simulink library "tqd"  (R2021b)
settings: Solver=VariableStepAuto  StartTime=0.0  StopTime=10.0  RelTol=1e-3
undefined symbols (not defined in the file or in its folder): ATQD_APSDecReq_X_kph, ATQD_APSDecReq_Y_mps2, ATQD_APSDecReqCMD_X_kph, ATQD_APSDecReqTs_X_pct, ATQD_APSDecTimeGain_X_Deg, ATQD_APSDecTimeGain_Y_s, ATQD_APSReqLowSpd_X_Deg, ATQD_AutoHoldReleaseBPS_X_Deg, ATQD_AWDLoadTrqnsGain_X_kg, ATQD_AWDLoadTrqnsGain_Y_pct, ATQD_BOSEnBPSPosn_X_kph, ATQD_BOSMap_X_rpm, ATQD_BOSMap_Y_pct, ATQD_CreepBaseTqD_X_kph, ATQD_CreepBaseTqD_Y_Deg, ATQD_CreepBaseTqR_X_kph, ATQD_CreepBaseTqR_Y_Deg, ATQD_CreepBPSDisPosn_X_Deg, ATQD_CreepBPSDisPosnR_X_Deg, ATQD_CreepBPSEnPosn_X_Deg, ATQD_CreepBPSEnPosnR_X_Deg, ATQD_CreepDeltaTq_X_kph, ATQD_CreepIterm_X_kph, ATQD_CreepIterm_Y_kph, ATQD_CreepItermMaxLimit_X_pct, ATQD_CreepPreloadTime_X_kph, ATQD_CreepPreloadTq_X_kph, ATQD_CreepPreloadTq_Y_s, ATQD_CreepProtTq_X_Deg, ATQD_CreepPterm_X_kph, ATQD_CreepPterm_Y_kph, ATQD_ECOTqMapD_X_rpm, ATQD_ECOTqMapD_Y_pct, ATQD_EOPDTqMapDCon_X_rpm, ATQD_EOPDTqMapDCon_Y_Deg, ATQD_EstInitVehWeight_X_c, ATQD_LHMRollGenMapD_X_rpm, ATQD_LHMRollGenMapD_Y_rpm, ATQD_LHMTqMapD_X_rpm, ATQD_LHMTqMapD_Y_pct, ATQD_NL1TqMapD_X_rpm, ATQD_NL1TqMapD_Y_pct, ATQD_NOPDTqMapDCon_X_rpm, ATQD_NOPDTqMapDCon_Y_Deg, ATQD_NRMRrEDUSpRat_X_rpm, ATQD_NRMRrEDUSpRat_Y_Nm, ATQD_OPDHoldDownRelDelay_X_Deg, ATQD_OPDHoldEnSpd_X_Deg, ATQD_OPDHoldRelDetTime_X_Deg, ATQD_OPDHoldReleaseTq_X_Deg, ATQD_OrigPedTqLowLim_X_Deg, ATQD_OrigPedTqLowLim_Y_pct, ATQD_PedalMapClimbUpLim_X_rpm, ATQD_PedalMapClimbUpLim_Y_Deg, ATQD_PreLoadTq_X_s, ATQD_RollGenMapEL1_X_rpm, ATQD_RollGenMapEL1_Y_rpm, ATQD_SL1TqMapD_X_rpm, ATQD_SL1TqMapD_Y_pct, ATQD_SlideRegenTqGain_X_Gps ... (+491)
libraries: hcu_lib x83, simulink x73, tqr x1
(part 3 of 19)

== system tqd/TQD/TorqueDemand/CrashDetect ==
  VPMM_PowerSta_enum : Inport
  VINP_CrashSignalGPIO_flg : Inport  Port=2
  VINP_CrashOutputSts_enum : Inport  Port=3
  task_time_s : Inport  Port=4
  Add1 : Sum
  Add2 : Sum
  Add3 : Sum
  Constant1 : Constant  Value=ENUM_POWERSTA_ON
  Constant{3,8,10,19,23,36} (6 alike) : Constant  Value=KTQD_CrashPWMCnt_cnt
  Constant{6,11,20,26,31,34} (6 alike) : Constant  Value=ZERO_INT
  Constant12 : Constant  Value=KTQD_50MS_cnt
  Constant13 : Constant  Value=KTQD_PwrStaTimerforCrash_s
  Constant14 : Constant  Value=ENUM_CRASHSTATE_NOCRASH
  Constant15 : Constant  Value=KTQD_DiagHCrashTimer_s
  Constant16 : Constant  Value=ENUM_CRASHSTATE_NOCRASH
  Constant17 : Constant  Value=ENUM_CRASHSTATE_NOCRASH
  Constant18 : Constant  Value=KTQD_PwrStaTimerforCrash_s
  Constant2 : Constant  Value=ENUM_POWERSTA_READY
  Constant21 : Constant  Value=KTQD_50MS_cnt
  Constant22 : Constant  Value=ZERO_FLOAT
  Constant24 : Constant  Value=KTQD_NoDiagHCrashTimer_s
  Constant25 : Constant  Value=KTQD_DiagHCrashTimer_s
  Constant27 : Constant  Value=KTQD_190MS_cnt
  Constant28 : Constant  Value=KTQD_30MS_cnt
  Constant29 : Constant  Value=KTQD_50MS_cnt
  Constant30 : Constant  Value=KTQD_210MS_cnt
  Constant32 : Constant  Value=KTQD_NoDiagHCrashTimer_s
  Constant35 : Constant  Value=KTQD_210MS_cnt
  Constant4 : Constant  Value=ONE_INT
  Constant5 : Constant  Value=ENUM_POWERSTA_OFF
  Constant7 : Constant  Value=KTQD_210MS_cnt
  Constant9 : Constant  Value=FALSE
  Data Type Conversion1 : DataTypeConversion
  Data Type Conversion2 : DataTypeConversion
  Equal : RelationalOperator  Operator=~=  OutDataTypeStr=boolean  RndMeth=Simplest
  Equal{1..2,6,10} (4 alike) : RelationalOperator  Operator===  OutDataTypeStr=boolean  RndMeth=Simplest
  Equal{3,7,9,11,13} (5 alike) : RelationalOperator  OutDataTypeStr=boolean  RndMeth=Simplest
  Equal12 : RelationalOperator  Operator=<  OutDataTypeStr=boolean  RndMeth=Simplest
  Equal4 : RelationalOperator  Operator=~=  OutDataTypeStr=boolean  RndMeth=Simplest
  Equal5 : RelationalOperator  Operator=<  OutDataTypeStr=boolean  RndMeth=Simplest
  Equal8 : RelationalOperator  Operator=~=  OutDataTypeStr=boolean  RndMeth=Simplest
  Logical Operator{,9..10,13,16,21} (6 alike) : Logic  Operator=OR  AllPortsSameDT=off  OutDataTypeStr=boolean
  Logical Operator{1,3,7..8,18,20} (6 alike) : Logic  Operator=NOT  AllPortsSameDT=off  OutDataTypeStr=boolean
  Logical Operator{4..5,11..12,14..15,17,19} (8 alike) : Logic  AllPortsSameDT=off  OutDataTypeStr=boolean
  Logical Operator2 : Logic  Inputs=3  AllPortsSameDT=off  OutDataTypeStr=boolean
  Logical Operator6 : Logic  Inputs=3  AllPortsSameDT=off  OutDataTypeStr=boolean
  Relational Operator{,5..7,9} (5 alike) : RelationalOperator  Operator=>  OutDataTypeStr=boolean  RndMeth=Simplest
  Relational Operator1 : RelationalOperator  OutDataTypeStr=boolean  RndMeth=Simplest
  Relational Operator10 : RelationalOperator  Operator=<  OutDataTypeStr=boolean  RndMeth=Simplest
  Relational Operator2 : RelationalOperator  Operator=<=  OutDataTypeStr=boolean  RndMeth=Simplest
  Relational Operator3 : RelationalOperator  OutDataTypeStr=boolean  RndMeth=Simplest
  Relational Operator4 : RelationalOperator  Operator=<=  OutDataTypeStr=boolean  RndMeth=Simplest
  Relational Operator8 : RelationalOperator  Operator=<  OutDataTypeStr=boolean  RndMeth=Simplest
  SR_Latch : hcu_lib/Basic_Blocks/SR_Latch
  Switch1 : Switch  Criteria=u2 ~= 0
  Switch{2..9} (8 alike) : Switch  Criteria=u2 > Threshold
  Timer2 : hcu_lib/Basic_Blocks/Timer
  Timer3 : hcu_lib/Basic_Blocks/Timer
  Timer4 : hcu_lib/Basic_Blocks/Timer
  Unit Delay{1..3,5} (4 alike) : UnitDelay  SampleTime=-1  HasFrameUpgradeWarning=on
  VTQD_CrashDetd_flg : Outport
  VTQD_DiagHCrash_flg : Outport  Port=2
  wires:
  [VPMM_PowerSta_enum] -> Equal2/1
  Logical Operator/1 -> Logical Operator3/1, Timer2/1
  [VPMM_PowerSta_enum] -> Equal1/1
  Constant13/1 -> Equal7/2
  Timer2/1 -> Equal7/1
  Constant18/1 -> Timer2/4
  Logical Operator3/1 -> Timer2/2
  Constant1/1 -> Equal1/2
  Constant2/1 -> Equal2/2
  Equal7/1 -> [VTQD_PwrStaTimerReady_flg]  "VTQD_PwrStaTimerReady_flg"
  [task_time_s] -> Timer2/3
  VPMM_PowerSta_enum/1 -> [VPMM_PowerSta_enum]
  VINP_CrashSignalGPIO_flg/1 -> [VINP_CrashSignalGPIO_flg]
  Equal1/1 -> Logical Operator/1
  Equal2/1 -> Logical Operator/2
  VINP_CrashOutputSts_enum/1 -> [VINP_CrashOutputSts_enum]
  task_time_s/1 -> [task_time_s]
  Data Type Conversion1/1 -> Add3/2
  Constant8/1 -> Relational Operator8/2
  Relational Operator8/1 -> Data Type Conversion1/1
  [VTQD_CrashCountEN_flg] -> Switch6/2
  [VTQD_PwrStaTimerReady_flg] -> Switch7/2
  Constant29/1 -> Relational Operator2/2
  Unit Delay3/1 -> Equal/1
  Constant26/1 -> Switch7/3
  Switch6/1 -> Switch3/1
  Logical Operator10/1 -> [VTQD_CrashCountEN_flg]
  Constant22/1 -> Relational Operator/2
  Add2/1 -> Switch2/3
  [VTQD_CrashChange_flg] -> Switch3/2
  Logical Operator6/1 -> Logical Operator10/2
  Constant28/1 -> Relational Operator1/2
  Logical Operator2/1 -> Logical Operator10/1
  Switch3/1 -> Switch7/1
  Equal/1 -> [VTQD_CrashChange_flg]
  Add3/1 -> Switch6/1
  Relational Operator3/1 -> Logical Operator6/2
  Constant6/1 -> Switch6/3
  Constant4/1 -> Add2/2
  Relational Operator2/1 -> Logical Operator2/3
  Logical Operator1/1 -> Logical Operator2/1
  [VTQD_fCrash_cnt] -> Relational Operator8/1, Add3/1
  Switch2/1 -> Unit Delay1/1
  Unit Delay5/1 -> [VTQD_fCrash_cnt], Equal3/1  "VTQD_fCrash_cnt"
  Relational Operator/1 -> Equal/2, Unit Delay3/1
  [VTQD_CrashChange_flg] -> Switch2/2
  [VINP_CrashSignalGPIO_flg] -> Logical Operator1/1
  [VTQD_CrashCount_enum] -> Relational Operator2/1, Relational Operator1/1
  Relational Operator1/1 -> Logical Operator2/2
  Constant31/1 -> Switch2/1
  [VINP_CrashSignalGPIO_flg] -> Relational Operator/1
  Constant10/1 -> Equal3/2
  [VTQD_PwrStaTimerReady_flg] -> Logical Operator12/2
  Logical Operator12/1 -> Logical Operator13/2, [VTQD_CrashOutputSts_flg]
  Equal4/1 -> Logical Operator12/1
  Constant14/1 -> Equal4/2
  [VINP_CrashOutputSts_enum] -> Equal4/1
  Switch7/1 -> Unit Delay5/1
  Unit Delay1/1 -> [VTQD_CrashCount_enum]
  [VTQD_CrashCount_enum] -> Add2/1
  Logical Operator4/1 -> Logical Operator9/2
  [VTQD_CrashCount_enum] -> Relational Operator6/1
  Relational Operator6/1 -> Logical Operator4/2
  [VINP_CrashSignalGPIO_flg] -> Logical Operator8/1
  Logical Operator5/1 -> Logical Operator9/1
  Constant7/1 -> Relational Operator6/2
  Constant11/1 -> Switch4/1
  Logical Operator8/1 -> Logical Operator4/1
  [VTQD_fCrash_cnt] -> Switch4/3
  [VTQD_CrashCount_enum] -> Relational Operator7/1
  Logical Operator9/1 -> Switch4/2
  Relational Operator7/1 -> Logical Operator5/2
  [VINP_CrashSignalGPIO_flg] -> Logical Operator5/1
  Constant12/1 -> Relational Operator7/2
  Switch4/1 -> Switch3/3
  Equal3/1 -> Logical Operator13/1
  Logical Operator13/1 -> VTQD_CrashDetd_flg/1  "VTQD_CrashDetd_flg"
  [VINP_CrashSignalGPIO_flg] -> Logical Operator6/1
  Relational Operator4/1 -> Logical Operator6/3
  Constant30/1 -> Relational Operator4/2
  Constant27/1 -> Relational Operator3/2
  [VTQD_CrashCount_enum] -> Relational Operator4/1, Relational Operator3/1
  [VINP_CrashSignalGPIO_flg] -> Logical Operator19/1
  Equal12/1 -> Logical Operator17/1
  Unit Delay2/1 -> Equal9/1, Equal12/1, [test_crash_cnt]
  Equal9/1 -> Logical Operator14/1
  [VINP_CrashOutputSts_enum] -> Equal8/1
  Data Type Conversion2/1 -> Add1/2
  [VTQD_CrashChange_flg] -> Switch5/2
  [test_crash_cnt] -> Relational Operator10/1, Add1/1
  Switch9/1 -> Switch5/1
  Logical Operator21/1 -> Switch8/2
  Constant15/1 -> Equal11/2
  Relational Operator5/1 -> Logical Operator15/2
  Equal6/1 -> Switch1/2
  Relational Operator10/1 -> Data Type Conversion2/1
  Constant34/1 -> Switch9/3
  [task_time_s] -> Timer4/3
  Logical Operator17/1 -> Logical Operator16/2
  Constant36/1 -> Relational Operator10/2
  SR_Latch/1 -> VTQD_DiagHCrash_flg/1  "VTQD_DiagHCrash_flg"
  Equal10/1 -> Logical Operator17/2
  Logical Operator20/1 -> Logical Operator15/1
  Constant20/1 -> Switch8/1
  Equal13/1 -> Switch1/3
  Relational Operator9/1 -> Logical Operator19/2
  Constant16/1 -> Equal8/2
  [VTQD_CrashCount_enum] -> Relational Operator9/1
  [VINP_CrashOutputSts_enum] -> Equal10/1
  Switch8/1 -> Switch5/3
  Equal11/1 -> Logical Operator11/2
  Logical Operator19/1 -> Logical Operator21/1
  Constant19/1 -> Equal9/2
  Constant21/1 -> Relational Operator9/2
  Constant17/1 -> Equal10/2
  Logical Operator18/1 -> Timer4/2
  [test_crash_cnt] -> Switch8/3
  Constant3/1 -> Equal5/2
  Logical Operator15/1 -> Logical Operator21/2
  Constant35/1 -> Relational Operator5/2
  Constant32/1 -> Timer4/4
  [VTQD_CrashCountEN_flg] -> Switch9/2
  Constant23/1 -> Equal12/2
  Equal8/1 -> Logical Operator14/2
  Constant24/1 -> Equal13/2
  [VPMM_PowerSta_enum] -> Equal6/1
  Add1/1 -> Switch9/1
  Logical Operator11/1 -> SR_Latch/1
  [VTQD_CrashOutputSts_flg] -> Logical Operator7/1, Timer3/1
  Switch1/1 -> SR_Latch/2
  Timer4/1 -> Equal13/1
  Constant9/1 -> Switch1/1
  [VINP_CrashSignalGPIO_flg] -> Logical Operator20/1
  [VTQD_fCrash_cnt] -> Equal5/1
  Logical Operator7/1 -> Timer3/2
  Switch5/1 -> Unit Delay2/1
  Equal5/1 -> Logical Operator11/1
  [task_time_s] -> Timer3/3
  Constant5/1 -> Equal6/2
  [VTQD_CrashCount_enum] -> Relational Operator5/1
  Constant25/1 -> Timer3/4
  Logical Operator16/1 -> Logical Operator18/1, Timer4/1
  Timer3/1 -> Equal11/1
  Logical Operator14/1 -> Logical Operator16/1

== system tqd/TQD/TorqueDemand/ShiftModule ==
  task_time_s : Inport
  VINP_ShifterHandleCmd_enum : Inport  Port=2
  VINP_VehSpeed_kph : Inport  Port=3
  VTQD_BrkSwSta_flg : Inport  Port=4
  VPMM_PowerSta_enum : Inport  Port=5
  VINP_PBWMotorPos_enum : Inport  Port=6
  VTQD_TMRotateDirction_enum : Inport  Port=7
  VTQD_EPBCarWashMode_flg : Inport  Port=8
  VINP_DrDoorSW_flg : Inport  Port=9
  VVMC_APSShiftPosnReq_enum : Inport  Port=10
  VVMC_APSActive_flg : Inport  Port=11
  VINP_DriverSeatBeltCmd_flg : Inport  Port=12
  VINP_SeatSW_flg : Inport  Port=13
  VINP_ChrgPlugSta_enum : Inport  Port=14
  VTQD_IVIPwrLock_flg : Inport  Port=15
  VTQD_AfterAvailableTqDemFr_Nm : Inport  Port=16
  VTQD_AfterAvailableTqDemRr_Nm : Inport  Port=17
  VTQR_NoABSFEDUWhlTqReq_Nm : Inport  Port=18
  VTQR_NoABSREDUWhlTqReq_Nm : Inport  Port=19
  VINP_DOASta_flg : Inport  Port=20
  VINP_MCPressure_bar : Inport  Port=21
  VTQD_OPDHoldAllowPark_flg : Inport  Port=22
  VINP_CAASSta_enum : Inport  Port=23
  VDDM_VCURAPSErrLv2_flg : Inport  Port=24
  VDDM_VCURAPSErrLv3_flg : Inport  Port=25
  VINP_APSStaSystem_enum : Inport  Port=26
  Constant : Constant  Value=KTQD_VehSpd2P_kph
  Constant1 : Constant  Value=KTQD_PBWTimeout_s
  Constant2 : Constant  Value=KTQD_VehSpdRev_kph
  Constant3 : Constant  Value=KTQD_ShiftInitialTime_s
  Constant4 : Constant  Value=KTQD_RelockWaitTime_s
  Constant5 : Constant  Value=KTQD_ReunlockWaitTime_s
  Constant6 : Constant  Value=ENUM_GEARACTUALPOSN_P
  Constant7 : Constant  Value=ENUM_GEARACTUALPOSN_P
  Data Type Conversion1 : DataTypeConversion
  Data Type Conversion2 : DataTypeConversion
  Data Type Conversion3 : DataTypeConversion  OutDataTypeStr=uint8
  Data Type Conversion4 : DataTypeConversion  OutDataTypeStr=boolean
  Determine_Actual_Gear_Position : Stateflow chart  TreatAsAtomicUnit=on
  Equal : RelationalOperator  Operator===  OutDataTypeStr=boolean  RndMeth=Simplest
  Equal1 : RelationalOperator  Operator=~=  OutDataTypeStr=boolean  RndMeth=Simplest
  GearShiftPosn : Subsystem  Description=GearPosition
  P_Button_State_Judge : Subsystem
  SR_Latch : hcu_lib/Basic_Blocks/SR_Latch
  SR_Latch1 : Subsystem  mask(SR_Latch){}
      mask help: SR latch function.
  VTQD_GearActualPosn_enum : Outport
  VTQD_ParkRequest_flg : Outport  Port=2
  VTQD_PBWLockTO_flg : Outport  Port=3
  VTQD_PBWUnlockTO_flg : Outport  Port=4
  VTQD_PButtonSta_enum : Outport  Port=5
  VTQD_DriveProtRemove_flg : Outport  Port=6
  VTQD_DriveProtEn_flg : Outport  Port=7
  wires:
  VPMM_PowerSta_enum/1 -> [VPMM_PowerSta_enum]
  task_time_s/1 -> [task_time_s]
  VINP_VehSpeed_kph/1 -> [VINP_VehSpeed_kph]
  VTQD_BrkSwSta_flg/1 -> [VTQD_BrkSwSta_flg]
  VTQD_TMRotateDirction_enum/1 -> [VTQD_TMRotateDirction_enum]
  VINP_PBWMotorPos_enum/1 -> [VINP_PBWMotorPos_enum]
  P_Button_State_Judge/1(VTQD_PButtonSta_enum) -> VTQD_PButtonSta_enum/1
  VINP_ShifterHandleCmd_enum/1 -> [VINP_ShifterHandleCmd_enum]
  [VINP_ShifterHandleCmd_enum] -> P_Button_State_Judge/1(VINP_ShifterHandleCmd_enum)
  VTQD_IVIPwrLock_flg/1 -> [VTQD_IVIPwrLock_flg]
  VINP_ChrgPlugSta_enum/1 -> [VINP_ChrgPlugSta_enum]
  VINP_SeatSW_flg/1 -> [VINP_SeatSW_flg]
  VINP_DriverSeatBeltCmd_flg/1 -> [VINP_DriverSeatBeltCmd_flg]
  VVMC_APSActive_flg/1 -> [VVMC_APSActive_flg]
  VVMC_APSShiftPosnReq_enum/1 -> [VVMC_APSShiftPosnReq_enum]
  VINP_DrDoorSW_flg/1 -> [VINP_DrDoorSW_flg]
  VTQD_EPBCarWashMode_flg/1 -> [VTQD_EPBCarWashMode_flg]
  [VTQD_EPBCarWashMode_flg] -> GearShiftPosn/8(VTQD_EPBCarWashMode_flg)
  [VINP_VehSpeed_kph] -> GearShiftPosn/9(VINP_VehSpeed_kph)
  [VINP_ChrgPlugSta_enum] -> GearShiftPosn/10(VINP_ChrgPlugSta_enum)
  GearShiftPosn/3(VTQD_PwrStaAllowDR_flg) -> [VTQD_PwrStaAllowDR_flg]
  [VVMC_APSShiftPosnReq_enum] -> GearShiftPosn/4(VVMC_APSShiftPosnReq_enum)
  [VINP_DrDoorSW_flg] -> GearShiftPosn/3(VINP_DrDoorSW_flg)
  [VINP_ShifterHandleCmd_enum] -> GearShiftPosn/1(VINP_ShifterHandleCmd_enum)
  [VVMC_APSActive_flg] -> GearShiftPosn/5(VVMC_APSActive_flg)
  [VINP_DriverSeatBeltCmd_flg] -> GearShiftPosn/6(VINP_DriverSeatBeltCmd_flg)
  GearShiftPosn/1(VTQD_GearShiftCMD_enum) -> [VTQD_GearShiftCMD_enum]
  [VINP_SeatSW_flg] -> GearShiftPosn/7(VINP_SeatSW_flg)
  [VPMM_PowerSta_enum] -> GearShiftPosn/2(VPMM_PowerSta_enum)
  GearShiftPosn/2(VTQD_PwrStaAllowPN_flg) -> [VTQD_PwrStaAllowPN_flg]
  [VVMC_APSActive_flg] -> Determine_Actual_Gear_Position/16(VVMC_APSActive_flg)
  Data Type Conversion4/1 -> VTQD_ParkRequest_flg/1  "VTQD_ParkRequest_flg"
  Constant6/1 -> Equal/2
  [VTQD_EPBCarWashMode_flg] -> Determine_Actual_Gear_Position/15(VINP_EPBCarWashMode_flg)
  Constant4/1 -> Determine_Actual_Gear_Position/13(KTQD_RelockWaitTime_s)
  Constant2/1 -> Determine_Actual_Gear_Position/10(KTQD_VehSpdRev_kph)
  Data Type Conversion1/1 -> SR_Latch/1
  [VTQD_GearActualPosn_enum] -> Equal1/1
  [VTQD_GearActualPosn_enum] -> Equal/1
  Data Type Conversion2/1 -> SR_Latch1/1(set)
  Determine_Actual_Gear_Position/4(VTQD_ParkRequest_flg) -> Data Type Conversion4/1
  Constant7/1 -> Equal1/2
  Data Type Conversion3/1 -> [VTQD_GearActualPosn_enum], VTQD_GearActualPosn_enum/1  "VTQD_GearActualPosn_enum"
  Constant1/1 -> Determine_Actual_Gear_Position/12(KTQD_PBWTimeout_s)
  Constant5/1 -> Determine_Actual_Gear_Position/14(KTQD_ReunlockWaitTime_s)
  [VTQD_PwrStaAllowPN_flg] -> Determine_Actual_Gear_Position/7(VTQD_PwrStaAllowPN_flg)
  Determine_Actual_Gear_Position/3(VTQD_PBWUnlockTO_flg) -> Data Type Conversion2/1
  Constant/1 -> Determine_Actual_Gear_Position/9(KTQD_VehSpd2P_kph)
  [VTQD_TMRotateDirction_enum] -> Determine_Actual_Gear_Position/8(VTQD_TMRotateDirction_enum)
  SR_Latch1/1(latched) -> VTQD_PBWUnlockTO_flg/1  "VTQD_PBWUnlockTO_flg"
  Equal1/1 -> SR_Latch1/2(reset)
  [VINP_VehSpeed_kph] -> Determine_Actual_Gear_Position/4(VINP_VehSpd_kph)
  [VTQD_PwrStaAllowDR_flg] -> Determine_Actual_Gear_Position/6(VTQD_PwrStaAllowDR_flg)
  Constant3/1 -> Determine_Actual_Gear_Position/11(KTQD_ShiftInitialTime_s)
  [VTQD_GearShiftCMD_enum] -> Determine_Actual_Gear_Position/3(VTQD_GearShiftCMD_enum)
  Equal/1 -> SR_Latch/2
  [task_time_s] -> Determine_Actual_Gear_Position/1(task_time_s)
  [VTQD_BrkSwSta_flg] -> Determine_Actual_Gear_Position/2(VTQD_BrkSwSta_flg)
  Determine_Actual_Gear_Position/2(VTQD_PBWLockTO_flg) -> Data Type Conversion1/1
  Determine_Actual_Gear_Position/1(VTQD_GearActualPosn_enum) -> Data Type Conversion3/1
  [VINP_PBWMotorPos_enum] -> Determine_Actual_Gear_Position/5(VINP_PBWMotorPos_enum)
  SR_Latch/1 -> VTQD_PBWLockTO_flg/1  "VTQD_PBWLockTO_flg"
  [VTQD_GearActualPosn_enum] -> GearShiftPosn/11(VTQD_GearActualPosn_enum)
  [VTQD_AfterAvailableTqDemFr_Nm] -> GearShiftPosn/12(VTQD_AfterAvailableTqDemFr_Nm)
  [VTQR_NoABSREDUWhlTqReq_Nm] -> GearShiftPosn/15(VTQR_NoABSREDUWhlTqReq_Nm)
  [VTQR_NoABSFEDUWhlTqReq_Nm] -> GearShiftPosn/14(VTQR_NoABSFEDUWhlTqReq_Nm)
  [VTQD_AfterAvailableTqDemRr_Nm] -> GearShiftPosn/13(VTQD_AfterAvailableTqDemRr_Nm)
  [task_time_s] -> GearShiftPosn/16(task_time_s)
  VTQD_AfterAvailableTqDemFr_Nm/1 -> [VTQD_AfterAvailableTqDemFr_Nm]
  VTQD_AfterAvailableTqDemRr_Nm/1 -> [VTQD_AfterAvailableTqDemRr_Nm]
  VTQR_NoABSFEDUWhlTqReq_Nm/1 -> [VTQR_NoABSFEDUWhlTqReq_Nm]
  VTQR_NoABSREDUWhlTqReq_Nm/1 -> [VTQR_NoABSREDUWhlTqReq_Nm]
  VINP_DOASta_flg/1 -> [VINP_DOASta_flg]
  [VINP_DOASta_flg] -> GearShiftPosn/17(VINP_DOASta_flg)
  GearShiftPosn/4(VTQD_DriveProtRemove_flg) -> VTQD_DriveProtRemove_flg/1
  GearShiftPosn/5(VTQD_DriveProtEn_flg) -> VTQD_DriveProtEn_flg/1
  [VTQD_IVIPwrLock_flg] -> GearShiftPosn/18(VTQD_IVIPwrLock_flg)
  [VTQD_BrkSwSta_flg] -> GearShiftPosn/19(VTQD_BrkSwSta_flg)
  GearShiftPosn/6(VTQD_ForceP_flg) -> [VTQD_ForceP_flg]
  [VTQD_ForceP_flg] -> Determine_Actual_Gear_Position/17(VTQD_ForceP_flg)
  VINP_MCPressure_bar/1 -> [VINP_MCPressure_bar]
  VTQD_OPDHoldAllowPark_flg/1 -> [VTQD_OPDHoldAllowPark_flg]
  [VTQD_OPDHoldAllowPark_flg] -> GearShiftPosn/20(VTQD_OPDHoldAllowPark_flg)
  VINP_CAASSta_enum/1 -> [VINP_CAASSta_enum]
  [VINP_CAASSta_enum] -> GearShiftPosn/21(VINP_CAASSta_enum)
  [VDDM_VCURAPSErrLv3_flg] -> GearShiftPosn/23(VDDM_VCURAPSErrLv3_flg)
  [VINP_APSStaSystem_enum] -> GearShiftPosn/24(VINP_APSStaSystem_enum)
  [VDDM_VCURAPSErrLv2_flg] -> GearShiftPosn/22(VDDM_VCURAPSErrLv2_flg)
  VDDM_VCURAPSErrLv3_flg/1 -> [VDDM_VCURAPSErrLv3_flg]
  VINP_APSStaSystem_enum/1 -> [VINP_APSStaSystem_enum]
  VDDM_VCURAPSErrLv2_flg/1 -> [VDDM_VCURAPSErrLv2_flg]
